simulink model "am_1"  (Simulink 4.00)
settings: Solver=ode45  StartTime=0  StopTime=1  RelTol=1e-3
undefined symbols (not defined in the file or in its folder): B, fn, Fs, get, k
libraries: dsparch3 x4, dspsnks3 x3, dspstat3 x3, dspmathops x3, commsource2 x1, dspsigattribs x1, dspbuff3 x1, dspspect3 x1
Description:
  | Model lacza cyfrowego z modulacja ASK/FSK/PSK
settings Model: Creator=Tomas  LimitDataPoints=off  MaxDataPoints=10000  RTWOptions="-aEnforceIntegerDowncast=1 -aExtMode=0 -aFoldNonRolledExpr=1 -aForceParamTrailComments=0 -aGenerateComments=1 -aIgnoreCustomStorageClasses=1 -aIncHierarchyInIds=0 -aInlineInvariantSignals=0 -aLocalBlockOutputs=1 -aLogVarNameModifier=\"rt_\" -aRTWVerbose=1 -aRollThreshold=5 -aShowEliminatedStatements=1"  RTWInlineParameters=on  BlockReductionOpt=off

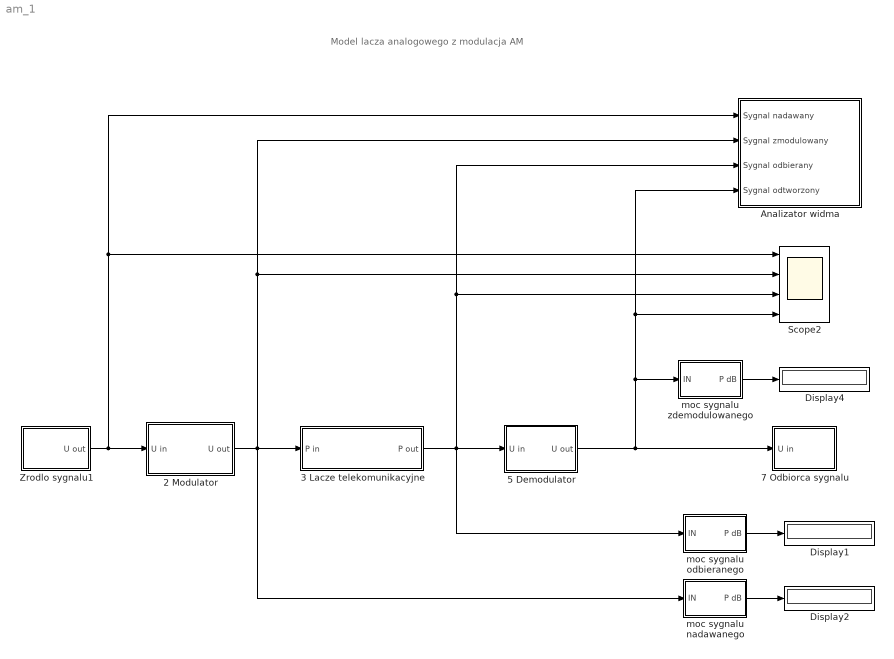
== system am_1 ==
  note: Model lacza analogowego z modulacja AM
  2 Modulator : Subsystem  mask(Modulator AM){on=on, p=0.7}
      mask prompts: on "Włączenie modulatora"; p "Głębokość modulacji (0..1):"
      mask help:
      | Dokonuje operacji modulacji AM sygnałem podanym na wejście.
      | Częstotliość nośnej: 1000 Hz.
      mask init:
      | fnos=1000;
      | if (on==0) k=1; set_param(gcb,'MaskEnables',{,'on','off'});
      | else set_param(gcb,'MaskEnables',{,'on','on'});
      |   if (p == 1) k = 0.1;
      |   elseif (p == 2) k = 0.2;
      |   elseif (p == 3) k = 0.3;
      |   elseif (p == 4) k = 0.4;
      |   elseif (p == 5) k = 0.5;
      |   elseif (p == 6) k = 0.6;
      |   elseif (p == 7) k = 0.7;
      |   elseif (p == 8) k = 0.8;
      |   elseif (p == 9) k = 0.9;
      |   elseif (p == 10) k = 1.0;
      |   else k = 1.5;
      |   end;
      | end;
      | on=on+1;
      settings: RTWFcnNameOpts=Auto  RTWFileNameOpts=Auto
      mask Help: No help
      mask StyleString: checkbox,popup(0.1|0.2|0.3|0.4|0.5|0.6|0.7|0.8|0.9|1.0|1.5)
      mask Display: disp('Modulator\nAM')
  "3 Lacze telekomunikacyjne " : Subsystem  mask(Łącze telekomunikacyjne){wn=off, sz=-30}
      mask prompts: wn "Dodanie szumu białego"; sz "Moc szumu [dB]:"
      mask help:
      | Filtruje i tłumi sygnał wejściowy według zadanych parametrów.
      | Na sygnał nakładany jest też szum biały wg rozkładu Gaussa.
      mask init:
      | sz=10^(sz/10);
      | if (wn == 0)
      | set_param(gcb,'MaskEnables',{,'on','off'});
      | else
      | set_param(gcb,'MaskEnables',{,'on','on'});
      | end;
      settings: RTWFcnNameOpts=Auto  RTWFileNameOpts=Auto
      mask Display: disp('Lacze \ntelekomunikacyjne')
  5 Demodulator : Subsystem  mask(Demodulator AM){typ=detektor synchroniczny, on=off, p=200}
      mask prompts: typ "Wybór typu demodulatora"; on "włącz filtr pasmowy"; p "pasmo filtru (Hz)"
      mask help:
      | Dokonuje operacji demodulacji AM sygnału podanego na wejście.
      | Częstotliwość nośnej: 1000 Hz.
      mask init:
      | fn=1000;
      | if (on==0) B=400; set_param(gcb,'MaskEnables',{,'on','on','off'});
      | else set_param(gcb,'MaskEnables',{,'on','on','on'});
      |   if (p == 1) B = 50;
      |   elseif (p == 2) B = 75;
      |   elseif (p == 3) B = 100;
      |   elseif (p == 4) B = 150;
      |   elseif (p == 5) B = 200;
      |   elseif (p == 6) B = 250;
      |   elseif (p == 7) B = 300;
      |   elseif (p == 8) B = 350;
      |   else B = 400;
      |   end;
      | B=16/15*B;
      | end;
      settings: RTWFcnNameOpts=Auto  RTWFileNameOpts=Auto
      mask Help: No help.
      mask StyleString: popup(detektor obwiedni|detektor synchroniczny),checkbox,popup(50|75|100|150|200|250|300|350|400)
      mask Display: disp('Demodulator\nAM')
  7 Odbiorca sygnalu : Subsystem
      settings: RTWFcnNameOpts=Auto  RTWFileNameOpts=Auto
      mask Type: Odbiorca sygnału
      mask Description: Odbiera sygnał przesylany od nadawcy.
      mask Help: No help
      mask Display: disp('Sygnal\nodbierany')
  "Analizator widma " : Subsystem
      settings: RTWFcnNameOpts=Auto  RTWFileNameOpts=Auto
  Display1 : Display
      settings: Format=short
  Display2 : Display
      settings: Format=short
  Display4 : Display
      settings: Format=short
  Scope2 : Scope  NumInputPorts=4
      settings: TimeRange=0.4  YMin=-1~-2.5~-2.5~0  YMax=1~2.5~2.5~1.75  SaveToWorkspace=off  SaveName=ScopeData  DataFormat=Array  MaxDataPoints=10000
  Zrodlo sygnalu1 : Subsystem  mask(Źródło sygnału){on=on, sq0=widmo płaskie 0..400Hz}
      mask prompts: on "Włączenie źródła sygnału"; sq0 "typ sygnału"
      mask help: Generuje sygnał źródłowy.
      mask init:
      | sq=sq0;
      | if (on == 0) set_param(gcb,'MaskEnables',{,'on','off'});
      | else set_param(gcb,'MaskEnables',{,'on','on'});
      | end;
      settings: RTWFcnNameOpts=Auto  RTWFileNameOpts=Auto
      mask Help: No help
      mask StyleString: checkbox,popup(f=100 Hz|widmo trójkątne 0..100Hz|widmo płaskie 0..100Hz|widmo płaskie 0..400Hz)
      mask Display: disp('Sygnal\nźródłowy')
  moc sygnalu zdemodulowanego : Subsystem  mask(Power dB){on=on}
      mask prompts: on "włącz"
      mask help: Oblicza w dB wartość mocy mierzonego sygnału
      settings: RTWFcnNameOpts=Auto  RTWFileNameOpts=Auto
  moc sygnalu nadawanego : Subsystem  mask(Power dB){on=on}
      mask prompts: on "włącz"
      mask help: Oblicza w dB wartość mocy mierzonego sygnału
      settings: RTWFcnNameOpts=Auto  RTWFileNameOpts=Auto
  moc sygnalu odbieranego : Subsystem  mask(Power dB){on=on}
      mask prompts: on "włącz"
      mask help: Oblicza w dB wartość mocy mierzonego sygnału
      settings: RTWFcnNameOpts=Auto  RTWFileNameOpts=Auto
  wires:
  Zrodlo sygnalu1/1(U out) -> Scope2/1, "Analizator widma "/1(Sygnal nadawany), 2 Modulator/1(U in)
  5 Demodulator/1(U out) -> Scope2/4, "Analizator widma "/4(Sygnal odtworzony), moc sygnalu zdemodulowanego/1(IN), 7 Odbiorca sygnalu/1(U in)
  2 Modulator/1(U out) -> Scope2/2, "Analizator widma "/2(Sygnal zmodulowany), "3 Lacze telekomunikacyjne "/1(P in), moc sygnalu nadawanego/1(IN)
  "3 Lacze telekomunikacyjne "/1(P out) -> Scope2/3, "Analizator widma "/3(Sygnal odbierany), 5 Demodulator/1(U in), moc sygnalu odbieranego/1(IN)
  moc sygnalu zdemodulowanego/1(P dB) -> Display4/1
  moc sygnalu odbieranego/1(P dB) -> Display1/1
  moc sygnalu nadawanego/1(P dB) -> Display2/1

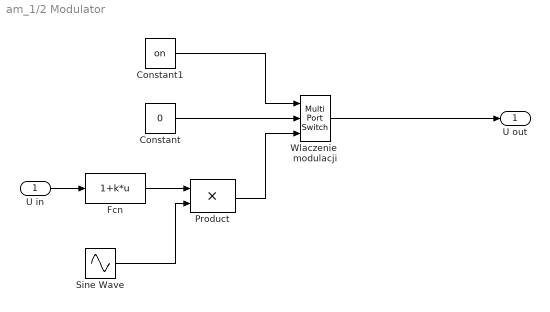
== system am_1/2 Modulator ==
  U in : Inport  Port=1  LatchInput=off
  Constant : Constant  Value=0
  Constant1 : Constant  Value=on
  Fcn : Fcn  Expr=1+k*u
  Product : Product  Inputs=2  Multiplication=Element-wise(.*)  SaturateOnIntegerOverflow=on
  Sine Wave : Sin  SineType=Time-based  Amplitude=1  Bias=0  Frequency=2*pi*1000  Phase=0  Samples=10  SampleTime=0  Offset=0
  Wlaczenie  modulacji : MultiPortSwitch  Inputs=2
  U out : Outport  Port=1
  wires:
  Wlaczenie  modulacji/1 -> U out/1
  Constant1/1 -> Wlaczenie  modulacji/1
  Constant/1 -> Wlaczenie  modulacji/2
  Product/1 -> Wlaczenie  modulacji/3
  U in/1 -> Fcn/1
  Fcn/1 -> Product/1
  Sine Wave/1 -> Product/2

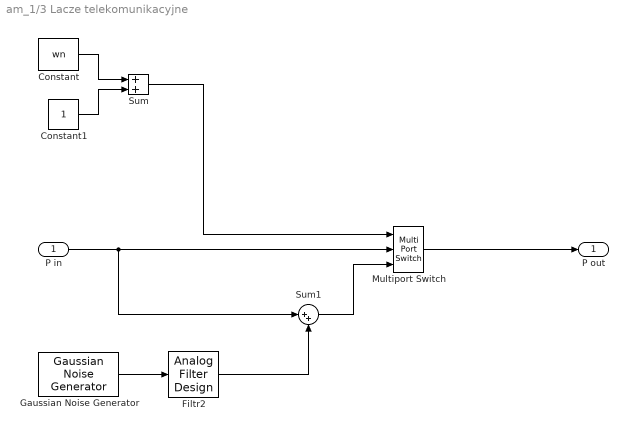
== system am_1/3 Lacze telekomunikacyjne  ==
  P in : Inport  Port=1  LatchInput=off
  Constant : Constant  Value=wn
  Constant1 : Constant  Value=1
  Filtr2 : dsparch3/Analog Filter Design  method=Butterworth  filttype=Lowpass  N=2  Wlo=2*pi*1000  Whi=2*pi*(fn+B/2)  Rp=2  Rs=40
  Gaussian Noise Generator : commsource2/Gaussian Noise Generator  m=0  d=sz/0.7333  s=12345  Ts=1/(6000)  frameBased=off  sampPerFrame=1  orient=off
  Multiport Switch : MultiPortSwitch  Inputs=2
  Sum : Sum  Inputs=++  SaturateOnIntegerOverflow=on
  Sum1 : Sum  Inputs=|++  SaturateOnIntegerOverflow=on
  P out : Outport  Port=1
  wires:
  P in/1 -> Sum1/1, Multiport Switch/2
  Constant/1 -> Sum/1
  Constant1/1 -> Sum/2
  Sum/1 -> Multiport Switch/1
  Multiport Switch/1 -> P out/1
  Sum1/1 -> Multiport Switch/3
  Gaussian Noise Generator/1 -> Filtr2/1
  Filtr2/1 -> Sum1/2

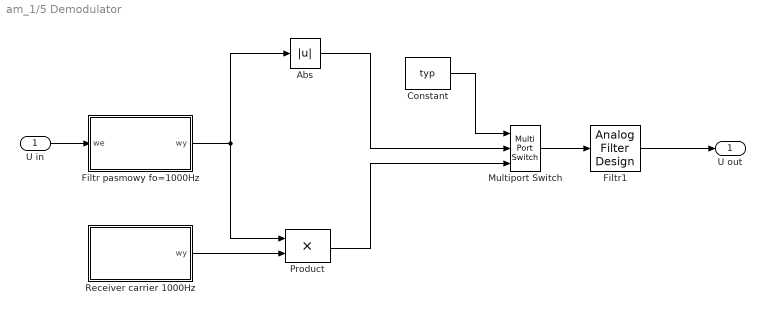
== system am_1/5 Demodulator ==
  U in : Inport  Port=1  LatchInput=off
  Abs : Abs  SaturateOnIntegerOverflow=on
  Constant : Constant  Value=typ
  Filtr pasmowy fo=1000Hz : Subsystem
      settings: RTWFcnNameOpts=Auto  RTWFileNameOpts=Auto
  Filtr1 : dsparch3/Analog Filter Design  method=Chebyshev II  filttype=Lowpass  N=16  Wlo=2*pi*(fn-B/2)  Whi=2*pi*(fn+B/2)  Rp=2  Rs=60
  Multiport Switch : MultiPortSwitch  Inputs=2
  Product : Product  Inputs=2  Multiplication=Element-wise(.*)  SaturateOnIntegerOverflow=on
  Receiver carrier 1000Hz : Subsystem
      settings: RTWFcnNameOpts=Auto  RTWFileNameOpts=Auto
  U out : Outport  Port=1
  wires:
  Multiport Switch/1 -> Filtr1/1
  Abs/1 -> Multiport Switch/2
  Constant/1 -> Multiport Switch/1
  Receiver carrier 1000Hz/1(wy) -> Product/2
  Product/1 -> Multiport Switch/3
  Filtr pasmowy fo=1000Hz/1(wy) -> Product/1, Abs/1
  U in/1 -> Filtr pasmowy fo=1000Hz/1(we)
  Filtr1/1 -> U out/1

== system am_1/7 Odbiorca sygnalu ==
  U in : Inport  Port=1  LatchInput=off
  Odbiorca : Terminator
  wires:
  U in/1 -> Odbiorca/1

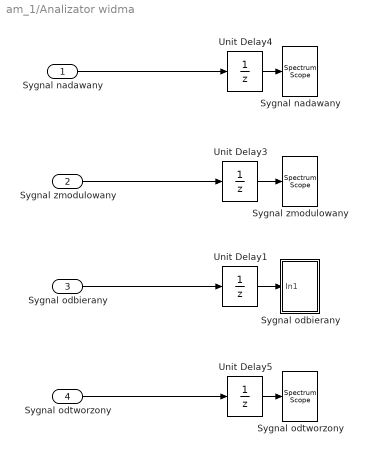
== system am_1/Analizator widma  ==
  Sygnal nadawany : Inport  Port=1  LatchInput=off
  Sygnal zmodulowany : Inport  Port=2  LatchInput=off
  Sygnal odbierany : Inport  Port=3  LatchInput=off
  Sygnal odtworzony : Inport  Port=4  LatchInput=off
  "Sygnal nadawany " : dspsnks3/Spectrum Scope  ScopeProperties=on  Domain=Frequency  HorizSpan=1  UseBuffer=on  BufferSize=4096  Overlap=0  inpFftLenInherit=off  FFTlength=128  numAvg=1  DisplayProperties=off  AxisGrid=on  Memory=on  FrameNumber=off  AxisLegend=off  AxisZoom=off  OpenScopeAtSimStart=on  OpenScopeImmediately=off  FigPos=get(0,'defaultfigureposition')  AxisProperties=off  XUnits=Hertz  XRange=[-Fs/2...Fs/2]  InheritXIncr=on  XIncr=1.0  XLabel=Samples  YUnits=dB  YLabel=Magnitude  LineProperties=off  LineMarkers=None
      settings: YMin=-10  YMax=23.8040697044832
  "Sygnal odtworzony " : dspsnks3/Spectrum Scope  ScopeProperties=on  Domain=Frequency  HorizSpan=1  UseBuffer=on  BufferSize=4096  Overlap=0  inpFftLenInherit=off  FFTlength=128  numAvg=1  DisplayProperties=off  AxisGrid=on  Memory=on  FrameNumber=off  AxisLegend=off  AxisZoom=off  OpenScopeAtSimStart=on  OpenScopeImmediately=off  FigPos=get(0,'defaultfigureposition')  AxisProperties=off  XUnits=Hertz  XRange=[-Fs/2...Fs/2]  InheritXIncr=on  XIncr=1.0  XLabel=Samples  YUnits=dB  YLabel=Magnitude  LineProperties=off  LineMarkers=None
      settings: YMin=-10  YMax=23.8040697044832
  "Sygnal zmodulowany " : dspsnks3/Spectrum Scope  ScopeProperties=on  Domain=Frequency  HorizSpan=1  UseBuffer=on  BufferSize=4096  Overlap=0  inpFftLenInherit=off  FFTlength=128  numAvg=1  DisplayProperties=off  AxisGrid=on  Memory=on  FrameNumber=off  AxisLegend=off  AxisZoom=off  OpenScopeAtSimStart=on  OpenScopeImmediately=off  FigPos=get(0,'defaultfigureposition')  AxisProperties=off  XUnits=Hertz  XRange=[-Fs/2...Fs/2]  InheritXIncr=on  XIncr=1.0  XLabel=Samples  YUnits=dB  YLabel=Magnitude  LineProperties=off  LineMarkers=None
      settings: YMin=-52.7531800625172  YMax=26.1007017107538
  "Sygnal odbierany " : Subsystem  AncestorBlock=dspsnks3/Spectrum Scope  TreatAsAtomicUnit=on  mask(Spectrum Scope){ScopeProperties=on, Domain=Frequency, HorizSpan=1, UseBuffer=on, BufferSize=4096, Overlap=0, inpFftLenInherit=off, FFTlength=128, numAvg=1, DisplayProperties=off, AxisGrid=on, Memory=on, FrameNumber=off, AxisLegend=off, AxisZoom=off, OpenScopeAtSimStart=on, OpenScopeImmediately=off, FigPos=get(0,'defaultfigureposition'), AxisProperties=off, XUnits=Hertz, XRange=[-Fs/2...Fs/2], InheritXIncr=on, XIncr=1.0, XLabel=Samples, YUnits=dB, YMin=-54.8494856104785, YMax=26.0788602500495, YLabel=Magnitude, LineProperties=off, LineDisables=, LineStyles=, LineMarkers=None, LineColors=}
      mask prompts: ScopeProperties "_______ Scope properties _______"; Domain "Input domain:"; HorizSpan "Time display span (number of frames):"; UseBuffer "Buffer input"; BufferSize "Buffer size:"; Overlap "Buffer overlap:"; inpFftLenInherit "Specify FFT length"; FFTlength "FFT length:"; numAvg "Number of spectral averages:"; DisplayProperties "_______ Display properties _______"; AxisGrid "Show grid"; Memory "Persistence"; FrameNumber "Frame number"; AxisLegend "Channel legend"; AxisZoom "Compact display"; OpenScopeAtSimStart "Open scope at start of simulation"; OpenScopeImmediately "Open scope immediately"; FigPos "Scope position:"; AxisProperties "_______ Axis properties _______"; XUnits "Frequency units:"; XRange "Frequency range:"; InheritXIncr "Inherit sample increment from input"; XIncr "Sample time of original time series:"; XLabel "X-axis title:"; YUnits "Amplitude scaling:"; YMin "Minimum Y-limit:"; YMax "Maximum Y-limit:"; YLabel "Y-axis title:"; LineProperties "_______ Line properties _______"; LineDisables "Line visibility:"; LineStyles "Line styles:"; LineMarkers "Line markers:"; LineColors "Line colors:"
      mask help: Compute and display the short-time FFT of each input signal. Non-frame based inputs to the block should use the buffering option.
      mask init:
      | [x,y,str] = dspblkbfftscope2('icon');
      | s = dspblkbfftscope2('init');
      settings: CopyFcn=sdspfscope2([],[],[],'BlockCopy');  DeleteFcn=sdspfscope2([],[],[],'BlockDelete');  NameChangeFcn=sdspfscope2([],[],[],'NameChange');  RTWSystemCode=Function  RTWFcnNameOpts=Auto  RTWFileNameOpts=Auto
      mask Help: web(dspbhelp);
      mask StyleString: checkbox,popup(Time|Frequency|User-defined),edit,checkbox,edit,edit,checkbox,edit,edit,checkbox,checkbox,checkbox,checkbox,checkbox,checkbox,checkbox,checkbox,edit,checkbox,popup(Hertz|rad/sec),popup([0...Fs/2]|[-Fs/2...Fs/2]|[0...Fs]),checkbox,edit,edit,popup(Magnitude|dB),edit,edit,edit,checkbox,edit,edit,edit,edit
      mask CallbackString: dspblkbfftscope2('dynamic','ScopeProperties')|||dspblkbfftscope2('dynamic','useBuffer');|||dspblkbfftscope2('dynamic','FftLenCheckbox');|||dspblkbfftscope2('dynamic','DisplayProperties');|||||||dspblkbfftscope2('dynamic','OpenScope');||dspblkbfftscope2('dynamic','AxisProperties');|||dspblkbfftscope2('dynamic','InheritXIncr');|||||||dspblkbfftscope2('dynamic','LineProperties');||||
      mask Display: plot(x,y); text(14,20,str);
  Unit Delay{1,3..5} (4 alike) : UnitDelay  X0=0  SampleTime=1/4096
      settings: RTWStateStorageClass=Auto
  wires:
  Unit Delay4/1 -> "Sygnal nadawany "/1
  Sygnal nadawany/1 -> Unit Delay4/1
  Unit Delay3/1 -> "Sygnal zmodulowany "/1
  Unit Delay5/1 -> "Sygnal odtworzony "/1
  Unit Delay1/1 -> "Sygnal odbierany "/1(In1)
  Sygnal zmodulowany/1 -> Unit Delay3/1
  Sygnal odbierany/1 -> Unit Delay1/1
  Sygnal odtworzony/1 -> Unit Delay5/1

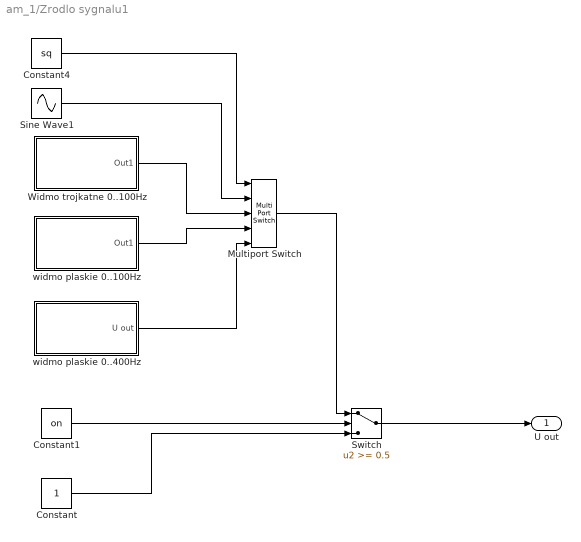
== system am_1/Zrodlo sygnalu1 ==
  Constant : Constant  Value=1
  Constant1 : Constant  Value=on
  Constant4 : Constant  Value=sq
  Multiport Switch : MultiPortSwitch  Inputs=4
  Sine Wave1 : Sin  SineType=Time-based  Amplitude=1  Bias=0  Frequency=2*pi*100  Phase=0  Samples=10  SampleTime=0  Offset=0
  Switch : Switch  Threshold=0.5
  Widmo trojkatne 0..100Hz : Subsystem
      settings: RTWFcnNameOpts=Auto  RTWFileNameOpts=Auto
  widmo plaskie 0..100Hz : Subsystem
      settings: RTWFcnNameOpts=Auto  RTWFileNameOpts=Auto
  widmo plaskie 0..400Hz : Subsystem
      settings: RTWFcnNameOpts=Auto  RTWFileNameOpts=Auto
  U out : Outport  Port=1
  wires:
  Switch/1 -> U out/1
  Constant/1 -> Switch/3
  Constant1/1 -> Switch/2
  Sine Wave1/1 -> Multiport Switch/2
  Multiport Switch/1 -> Switch/1
  Constant4/1 -> Multiport Switch/1
  Widmo trojkatne 0..100Hz/1(Out1) -> Multiport Switch/3
  widmo plaskie 0..100Hz/1(Out1) -> Multiport Switch/4
  widmo plaskie 0..400Hz/1(U out) -> Multiport Switch/5

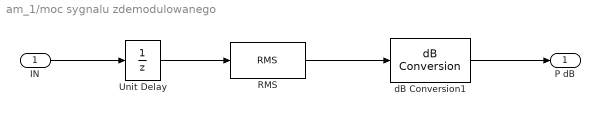
== system am_1/moc sygnalu zdemodulowanego ==
  IN : Inport  Port=1  LatchInput=off
  RMS : dspstat3/RMS  run=on  reset_popup=None
  Unit Delay : UnitDelay  X0=0  SampleTime=1/2048
      settings: RTWStateStorageClass=Auto
  dB Conversion1 : dspmathops/dB Conversion  dBtype=dB  intype=Amplitude  R=1  fuzz=on
  P dB : Outport  Port=1
  wires:
  dB Conversion1/1 -> P dB/1
  RMS/1 -> dB Conversion1/1
  IN/1 -> Unit Delay/1
  Unit Delay/1 -> RMS/1

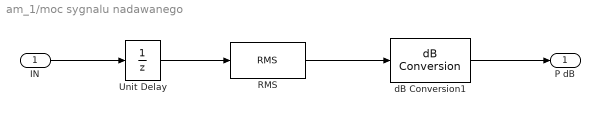
== system am_1/moc sygnalu nadawanego ==
  IN : Inport  Port=1  LatchInput=off
  RMS : dspstat3/RMS  run=on  reset_popup=None
  Unit Delay : UnitDelay  X0=0  SampleTime=1/4096
      settings: RTWStateStorageClass=Auto
  dB Conversion1 : dspmathops/dB Conversion  dBtype=dB  intype=Amplitude  R=1  fuzz=on
  P dB : Outport  Port=1
  wires:
  dB Conversion1/1 -> P dB/1
  RMS/1 -> dB Conversion1/1
  IN/1 -> Unit Delay/1
  Unit Delay/1 -> RMS/1

== system am_1/moc sygnalu odbieranego ==
  IN : Inport  Port=1  LatchInput=off
  RMS : dspstat3/RMS  run=on  reset_popup=None
  Unit Delay : UnitDelay  X0=0  SampleTime=1/4096
      settings: RTWStateStorageClass=Auto
  dB Conversion1 : dspmathops/dB Conversion  dBtype=dB  intype=Amplitude  R=1  fuzz=on
  P dB : Outport  Port=1
  wires:
  dB Conversion1/1 -> P dB/1
  RMS/1 -> dB Conversion1/1
  IN/1 -> Unit Delay/1
  Unit Delay/1 -> RMS/1

== system am_1/5 Demodulator/Filtr pasmowy fo=1000Hz ==
  we : Inport  Port=1  LatchInput=off
  Constant2 : Constant  Value=on
  Filtr2 : dsparch3/Analog Filter Design  method=Chebyshev II  filttype=Bandpass  N=20  Wlo=2*pi*(fn-B/2)  Whi=2*pi*(fn+B/2)  Rp=2  Rs=60
  Switch3 : Switch  Threshold=0.5
  wy : Outport  Port=1
  wires:
  we/1 -> Filtr2/1, Switch3/3
  Constant2/1 -> Switch3/2
  Filtr2/1 -> Switch3/1
  Switch3/1 -> wy/1

== system am_1/5 Demodulator/Receiver carrier 1000Hz ==
  Constant2 : Constant  Value=on
  Filtr2 : dsparch3/Analog Filter Design  method=Chebyshev II  filttype=Bandpass  N=20  Wlo=2*pi*(fn-B/2)  Whi=2*pi*(fn+B/2)  Rp=2  Rs=60
  Sine Wave : Sin  SineType=Time-based  Amplitude=1  Bias=0  Frequency=2*pi*fn  Phase=0  Samples=10  SampleTime=0  Offset=0
  Switch3 : Switch  Threshold=0.5
  wy : Outport  Port=1
  wires:
  Sine Wave/1 -> Filtr2/1, Switch3/3
  Constant2/1 -> Switch3/2
  Filtr2/1 -> Switch3/1
  Switch3/1 -> wy/1

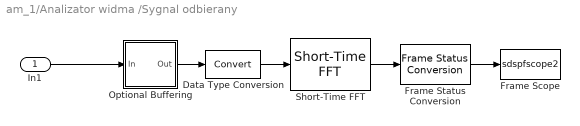
== system am_1/Analizator widma /Sygnal odbierany  ==
  In1 : Inport  Port=1  LatchInput=off
  Data Type Conversion : DataTypeConversion  DataType=double  SaturateOnIntegerOverflow=on
  Frame Scope : S-Function  FunctionName=sdspfscope2  Parameters=s  PortCounts=[]  SFunctionModules=''
  Frame Status Conversion : dspsigattribs/Frame Status Conversion  growRefPort=off  outframe=Sample-based
  Optional Buffering : Subsystem  mask(Replaceable Contents){oname=Buffer, osrc=dspbuff3/Buffer, oargs={'N','BufferSize','V','Overlap','ic','0'}, replace=strcmp(UseBuffer,'off')}
      mask prompts: oname "Relative name of blocks to replace:"; osrc "Simulink path to each source block:"; oargs "Parameter/value pairs to each block:"; replace "Replace with short-circuit:"
      mask help: Configurable subsystem holding blocks which may be replaced by virtual short-circuits (muxes) when not needed.
      mask init:
      | opts.name = oname; opts.src = osrc; opts.args = oargs;
      | dspskipblk(gcb,opts,replace);
      settings: RTWFcnNameOpts=Auto  RTWFileNameOpts=Auto
  Short-Time FFT : dspspect3/Short-Time FFT  wintype=Hann  Rs=50  beta=5  winsamp=Symmetric  inheritFFT=on  fftsize=FFTlength  navg=numAvg
  wires:
  Data Type Conversion/1 -> Short-Time FFT/1
  Optional Buffering/1(Out) -> Data Type Conversion/1
  Short-Time FFT/1 -> Frame Status Conversion/1
  Frame Status Conversion/1 -> Frame Scope/1
  In1/1 -> Optional Buffering/1(In)

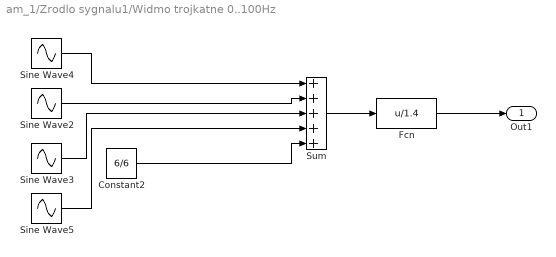
== system am_1/Zrodlo sygnalu1/Widmo trojkatne 0..100Hz ==
  Constant2 : Constant  Value=6/6
  Fcn : Fcn  Expr=u/1.4
  Sine Wave2 : Sin  SineType=Time-based  Amplitude=1.5/6  Bias=0  Frequency=2*pi*50  Phase=0  Samples=10  SampleTime=0  Offset=0
  Sine Wave3 : Sin  SineType=Time-based  Amplitude=0.5/6  Bias=0  Frequency=2*pi*75  Phase=0  Samples=10  SampleTime=0  Offset=0
  Sine Wave4 : Sin  SineType=Time-based  Amplitude=3/6  Bias=0  Frequency=2*pi*25  Phase=0  Samples=10  SampleTime=0  Offset=0
  Sine Wave5 : Sin  SineType=Time-based  Amplitude=0.5/3/6  Bias=0  Frequency=2*pi*100  Phase=0  Samples=10  SampleTime=0  Offset=0
  Sum : Sum  Inputs=5  SaturateOnIntegerOverflow=on
  Out1 : Outport  Port=1
  wires:
  Sine Wave4/1 -> Sum/1
  Sine Wave2/1 -> Sum/2
  Sine Wave3/1 -> Sum/3
  Sine Wave5/1 -> Sum/4
  Constant2/1 -> Sum/5
  Sum/1 -> Fcn/1
  Fcn/1 -> Out1/1

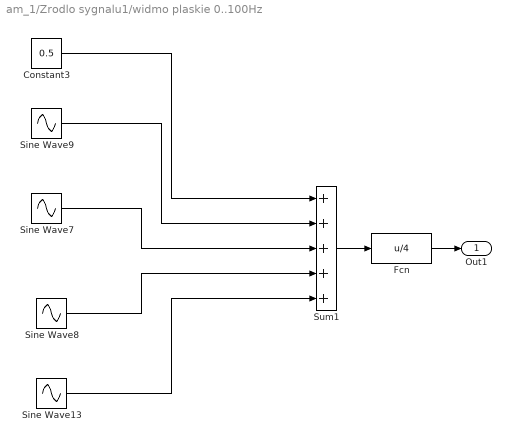
== system am_1/Zrodlo sygnalu1/widmo plaskie 0..100Hz ==
  Constant3 : Constant  Value=0.5
  Fcn : Fcn  Expr=u/4
  Sine Wave13 : Sin  SineType=Time-based  Amplitude=1  Bias=0  Frequency=2*pi*100  Phase=0  Samples=10  SampleTime=0  Offset=0
  Sine Wave7 : Sin  SineType=Time-based  Amplitude=1  Bias=0  Frequency=2*pi*50  Phase=0  Samples=10  SampleTime=0  Offset=0
  Sine Wave8 : Sin  SineType=Time-based  Amplitude=1  Bias=0  Frequency=2*pi*75  Phase=0  Samples=10  SampleTime=0  Offset=0
  Sine Wave9 : Sin  SineType=Time-based  Amplitude=1  Bias=0  Frequency=2*pi*25  Phase=0  Samples=10  SampleTime=0  Offset=0
  Sum1 : Sum  Inputs=5  SaturateOnIntegerOverflow=on
  Out1 : Outport  Port=1
  wires:
  Sine Wave9/1 -> Sum1/2
  Sine Wave7/1 -> Sum1/3
  Sine Wave8/1 -> Sum1/4
  Sine Wave13/1 -> Sum1/5
  Constant3/1 -> Sum1/1
  Sum1/1 -> Fcn/1
  Fcn/1 -> Out1/1

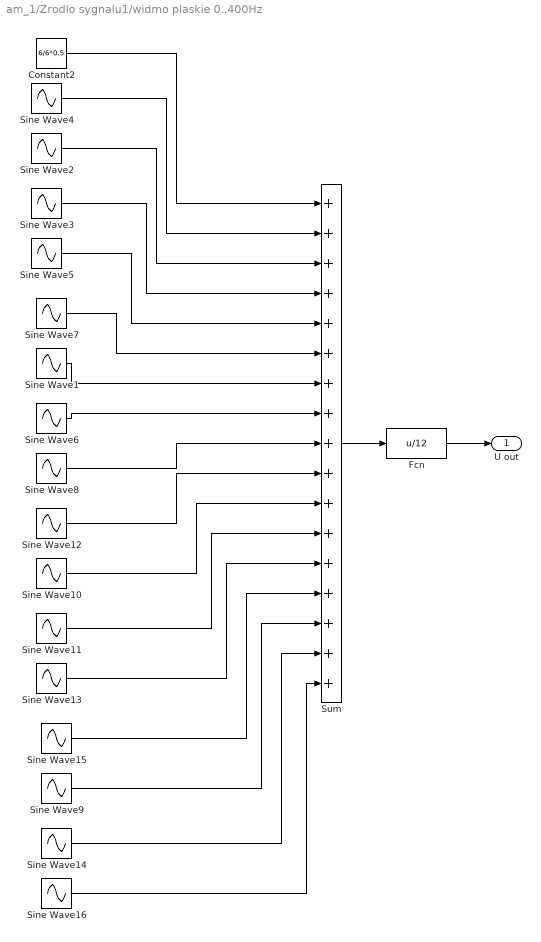
== system am_1/Zrodlo sygnalu1/widmo plaskie 0..400Hz ==
  Constant2 : Constant  Value=6/6*0.5
  Fcn : Fcn  Expr=u/12
  Sine Wave1 : Sin  SineType=Time-based  Amplitude=1  Bias=0  Frequency=2*pi*150  Phase=0  Samples=10  SampleTime=0  Offset=0
  Sine Wave10 : Sin  SineType=Time-based  Amplitude=1  Bias=0  Frequency=2*pi*250  Phase=0  Samples=10  SampleTime=0  Offset=0
  Sine Wave11 : Sin  SineType=Time-based  Amplitude=1  Bias=0  Frequency=2*pi*275  Phase=0  Samples=10  SampleTime=0  Offset=0
  Sine Wave12 : Sin  SineType=Time-based  Amplitude=1  Bias=0  Frequency=2*pi*225  Phase=0  Samples=10  SampleTime=0  Offset=0
  Sine Wave13 : Sin  SineType=Time-based  Amplitude=1  Bias=0  Frequency=2*pi*300  Phase=0  Samples=10  SampleTime=0  Offset=0
  Sine Wave14 : Sin  SineType=Time-based  Amplitude=1  Bias=0  Frequency=2*pi*375  Phase=0  Samples=10  SampleTime=0  Offset=0
  Sine Wave15 : Sin  SineType=Time-based  Amplitude=1  Bias=0  Frequency=2*pi*325  Phase=0  Samples=10  SampleTime=0  Offset=0
  Sine Wave16 : Sin  SineType=Time-based  Amplitude=1  Bias=0  Frequency=2*pi*400  Phase=0  Samples=10  SampleTime=0  Offset=0
  Sine Wave2 : Sin  SineType=Time-based  Amplitude=1  Bias=0  Frequency=2*pi*50  Phase=0  Samples=10  SampleTime=0  Offset=0
  Sine Wave3 : Sin  SineType=Time-based  Amplitude=1  Bias=0  Frequency=2*pi*75  Phase=0  Samples=10  SampleTime=0  Offset=0
  Sine Wave4 : Sin  SineType=Time-based  Amplitude=1  Bias=0  Frequency=2*pi*25  Phase=0  Samples=10  SampleTime=0  Offset=0
  Sine Wave5 : Sin  SineType=Time-based  Amplitude=1  Bias=0  Frequency=2*pi*100  Phase=0  Samples=10  SampleTime=0  Offset=0
  Sine Wave6 : Sin  SineType=Time-based  Amplitude=1  Bias=0  Frequency=2*pi*175  Phase=0  Samples=10  SampleTime=0  Offset=0
  Sine Wave7 : Sin  SineType=Time-based  Amplitude=1  Bias=0  Frequency=2*pi*125  Phase=0  Samples=10  SampleTime=0  Offset=0
  Sine Wave8 : Sin  SineType=Time-based  Amplitude=1  Bias=0  Frequency=2*pi*200  Phase=0  Samples=10  SampleTime=0  Offset=0
  Sine Wave9 : Sin  SineType=Time-based  Amplitude=1  Bias=0  Frequency=2*pi*350  Phase=0  Samples=10  SampleTime=0  Offset=0
  Sum : Sum  Inputs=17  SaturateOnIntegerOverflow=on
  U out : Outport  Port=1
  wires:
  Sine Wave4/1 -> Sum/2
  Sine Wave2/1 -> Sum/3
  Sine Wave3/1 -> Sum/4
  Sine Wave5/1 -> Sum/5
  Constant2/1 -> Sum/1
  Sine Wave7/1 -> Sum/6
  Sine Wave1/1 -> Sum/7
  Sine Wave6/1 -> Sum/8
  Sine Wave8/1 -> Sum/9
  Sine Wave12/1 -> Sum/10
  Sine Wave10/1 -> Sum/11
  Sine Wave11/1 -> Sum/12
  Sine Wave13/1 -> Sum/13
  Sine Wave15/1 -> Sum/14
  Sine Wave9/1 -> Sum/15
  Sine Wave14/1 -> Sum/16
  Sine Wave16/1 -> Sum/17
  Sum/1 -> Fcn/1
  Fcn/1 -> U out/1

== system am_1/Analizator widma /Sygnal odbierany /Optional Buffering ==
  In : Inport  Port=1  LatchInput=off
  Buffer : dspbuff3/Buffer  N=BufferSize  V=Overlap  ic=0
  Out : Outport  Port=1  InitialOutput=0
  wires:
  In/1 -> Buffer/1
  Buffer/1 -> Out/1
